simulink library "csu_egm_estimated_gravity_model_lib"  (R2014b)
settings: Solver=ode45  StartTime=0.0  StopTime=10.0  RelTol=1e-3
undefined symbols (not defined in the file or in its folder): central_body_flattening, central_body_gravity_mu, gsh_a, gsh_b, gsh_e, gsh_ep, magnitude
libraries: util_quat_lib x7, util_common_lib x3, util_fsw_frame_rotation_lib x2
settings Model: Creator=escrane  LastModifiedBy=escrane

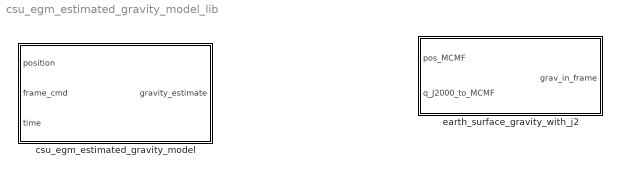
== system csu_egm_estimated_gravity_model_lib ==
  csu_egm_estimated_gravity_model : Subsystem
  earth_surface_gravity_with_j2 : Subsystem

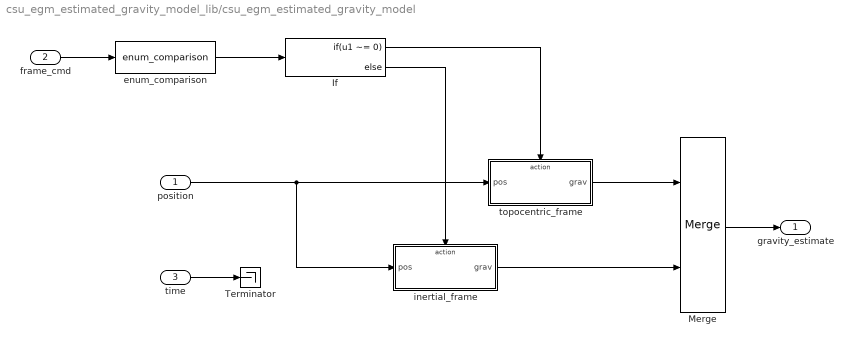
== system csu_egm_estimated_gravity_model_lib/csu_egm_estimated_gravity_model ==
  position : Inport
  frame_cmd : Inport  Port=2
  time : Inport  Port=3
  If : If  IfExpression=u1 ~= 0
  Merge : Merge
  Terminator : Terminator
  enum_comparison : util_common_lib/enum_comparison  comparison_type===
  inertial_frame : Subsystem
  topocentric_frame : Subsystem
  gravity_estimate : Outport
  wires:
  position/1 -> inertial_frame/1(pos), topocentric_frame/1(pos)
  frame_cmd/1 -> enum_comparison/1
  enum_comparison/1 -> If/1
  If/1 -> topocentric_frame/Action
  If/2 -> inertial_frame/Action
  topocentric_frame/1(grav) -> Merge/1
  inertial_frame/1(grav) -> Merge/2
  Merge/1 -> gravity_estimate/1
  time/1 -> Terminator/1

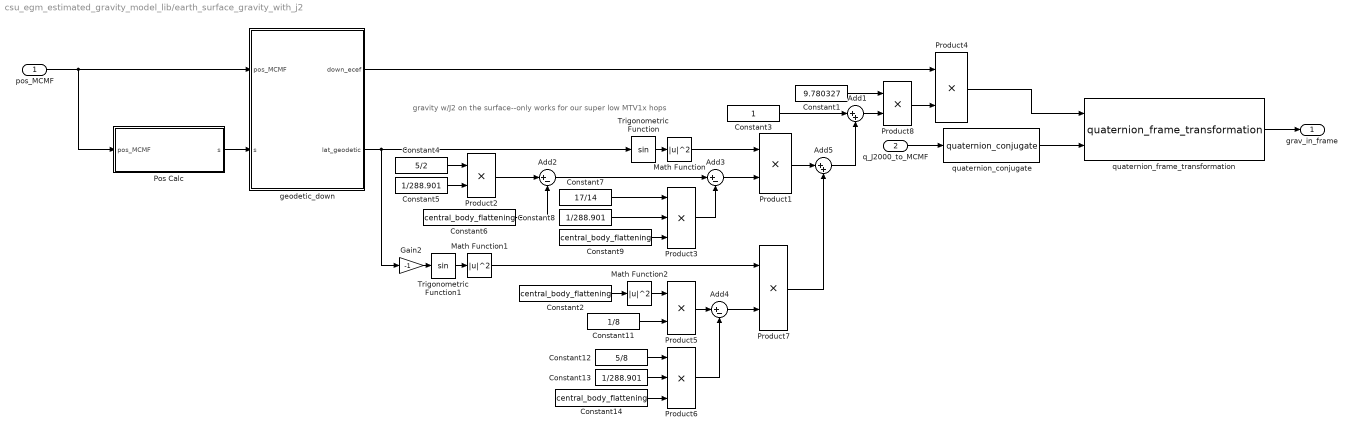
== system csu_egm_estimated_gravity_model_lib/earth_surface_gravity_with_j2 ==
  note: gravity w/J2 on the surface--only works for our super low MTV1x hops
  pos_MCMF : Inport
  q_J2000_to_MCMF : Inport  Port=2
  Add1 : Sum  Inputs=|++
  Add2 : Sum  Inputs=|+-
  Add3 : Sum  Inputs=|+-
  Add4 : Sum  Inputs=|+-
  Add5 : Sum  Inputs=|++
  Constant1 : Constant  Value=9.780327
  Constant11 : Constant  Value=1/8
  Constant12 : Constant  Value=5/8
  Constant13 : Constant  Value=1/288.901
  Constant{2,6,9,14} (4 alike) : Constant  Value=central_body_flattening
  Constant3 : Constant
  Constant4 : Constant  Value=5/2
  Constant5 : Constant  Value=1/288.901
  Constant7 : Constant  Value=17/14
  Constant8 : Constant  Value=1/288.901
  Gain2 : Gain  Gain=-1
  Math Function : Math  Operator=magnitude^2  SaturateOnIntegerOverflow=on
  Math Function1 : Math  Operator=magnitude^2  SaturateOnIntegerOverflow=on
  Math Function2 : Math  Operator=magnitude^2  SaturateOnIntegerOverflow=on
  Pos Calc : Subsystem
  Product{1..2,4..5,7..8} (6 alike) : Product
  Product3 : Product  Inputs=3
  Product6 : Product  Inputs=3
  Trigonometric Function : Trigonometry
  Trigonometric Function1 : Trigonometry
  geodetic_down : Subsystem
  quaternion_conjugate : util_quat_lib/quaternion_conjugate  SystemSampleTime=-1
  quaternion_frame_transformation : util_quat_lib/quaternion_frame_transformation  SystemSampleTime=-1
  grav_in_frame : Outport
  wires:
  quaternion_frame_transformation/1 -> grav_in_frame/1
  Product4/1 -> quaternion_frame_transformation/1
  quaternion_conjugate/1 -> quaternion_frame_transformation/2
  q_J2000_to_MCMF/1 -> quaternion_conjugate/1
  Pos Calc/1(s) -> geodetic_down/2(s)
  pos_MCMF/1 -> Pos Calc/1(pos_MCMF), geodetic_down/1(pos_MCMF)
  Constant3/1 -> Add1/1
  Trigonometric Function/1 -> Math Function/1
  Trigonometric Function1/1 -> Math Function1/1
  geodetic_down/2(lat_geodetic) -> Gain2/1, Trigonometric Function/1
  Gain2/1 -> Trigonometric Function1/1
  Constant4/1 -> Product2/1
  Constant5/1 -> Product2/2
  Product2/1 -> Add2/1
  Constant6/1 -> Add2/2
  Constant7/1 -> Product3/1
  Constant8/1 -> Product3/2
  Constant9/1 -> Product3/3
  Add2/1 -> Add3/1
  Product3/1 -> Add3/2
  Math Function/1 -> Product1/1
  Add3/1 -> Product1/2
  Constant2/1 -> Math Function2/1
  Math Function2/1 -> Product5/1
  Constant11/1 -> Product5/2
  Constant12/1 -> Product6/1
  Constant13/1 -> Product6/2
  Constant14/1 -> Product6/3
  Product5/1 -> Add4/1
  Product6/1 -> Add4/2
  Add4/1 -> Product7/2
  Math Function1/1 -> Product7/1
  Product1/1 -> Add5/1
  Product7/1 -> Add5/2
  Add5/1 -> Add1/2
  Add1/1 -> Product8/2
  Constant1/1 -> Product8/1
  Product8/1 -> Product4/2
  geodetic_down/1(down_ecef) -> Product4/1

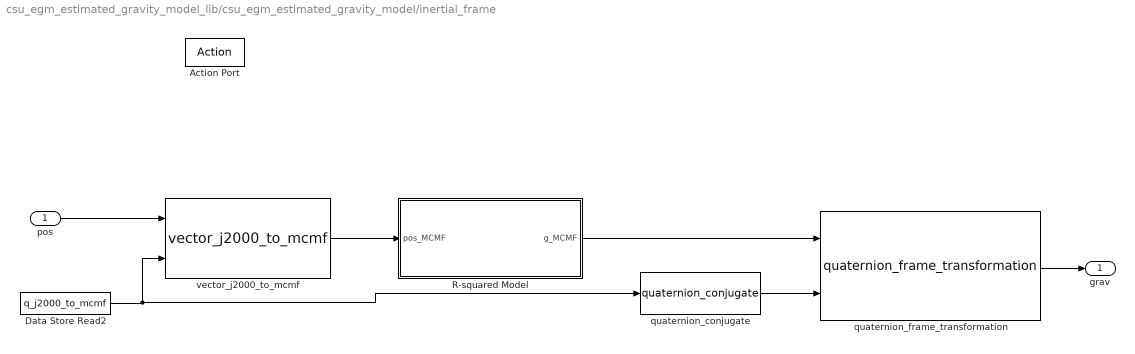
== system csu_egm_estimated_gravity_model_lib/csu_egm_estimated_gravity_model/inertial_frame ==
  pos : Inport
  Action Port : ActionPort
  Data Store Read2 : DataStoreRead  DataStoreName=q_j2000_to_mcmf
  R-squared Model : Subsystem
  quaternion_conjugate : util_quat_lib/quaternion_conjugate  SystemSampleTime=-1
  quaternion_frame_transformation : util_quat_lib/quaternion_frame_transformation  SystemSampleTime=-1
  vector_j2000_to_mcmf : util_fsw_frame_rotation_lib/vector_j2000_to_mcmf  SystemSampleTime=-1
  grav : Outport
  wires:
  R-squared Model/1(g_MCMF) -> quaternion_frame_transformation/1
  quaternion_conjugate/1 -> quaternion_frame_transformation/2
  pos/1 -> vector_j2000_to_mcmf/1
  quaternion_frame_transformation/1 -> grav/1
  Data Store Read2/1 -> vector_j2000_to_mcmf/2, quaternion_conjugate/1
  vector_j2000_to_mcmf/1 -> R-squared Model/1(pos_MCMF)

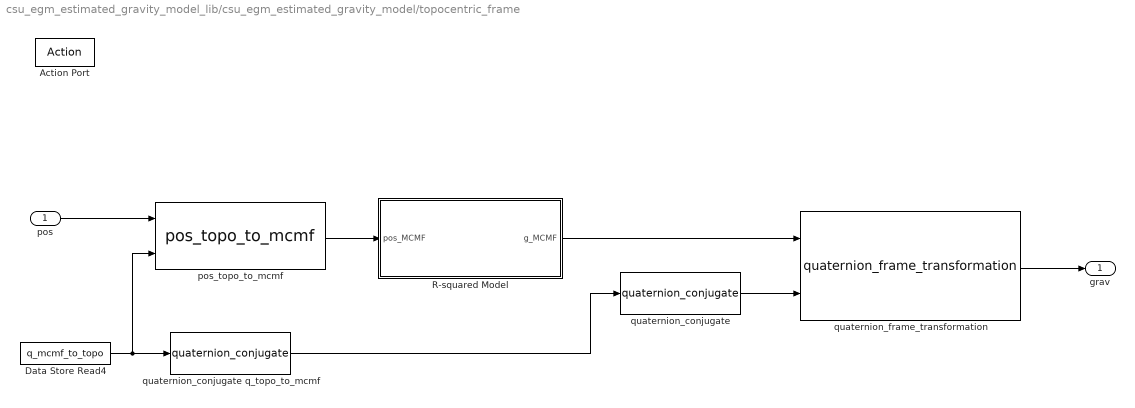
== system csu_egm_estimated_gravity_model_lib/csu_egm_estimated_gravity_model/topocentric_frame ==
  pos : Inport
  Action Port : ActionPort
  Data Store Read4 : DataStoreRead  DataStoreName=q_mcmf_to_topo
  R-squared Model : Subsystem
  pos_topo_to_mcmf : util_fsw_frame_rotation_lib/pos_topo_to_mcmf  SystemSampleTime=-1
  quaternion_conjugate : util_quat_lib/quaternion_conjugate  SystemSampleTime=-1
  quaternion_conjugate q_topo_to_mcmf : util_quat_lib/quaternion_conjugate  SystemSampleTime=-1
  quaternion_frame_transformation : util_quat_lib/quaternion_frame_transformation  SystemSampleTime=-1
  grav : Outport
  wires:
  R-squared Model/1(g_MCMF) -> quaternion_frame_transformation/1
  quaternion_conjugate/1 -> quaternion_frame_transformation/2
  quaternion_frame_transformation/1 -> grav/1
  pos_topo_to_mcmf/1 -> R-squared Model/1(pos_MCMF)
  pos/1 -> pos_topo_to_mcmf/1
  Data Store Read4/1 -> quaternion_conjugate q_topo_to_mcmf/1, pos_topo_to_mcmf/2
  quaternion_conjugate q_topo_to_mcmf/1 -> quaternion_conjugate/1

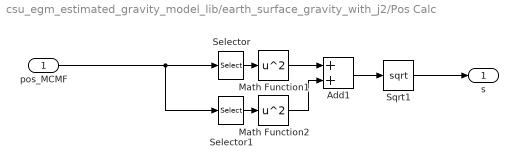
== system csu_egm_estimated_gravity_model_lib/earth_surface_gravity_with_j2/Pos Calc ==
  pos_MCMF : Inport
  Add1 : Sum
  Math Function1 : Math  Operator=square  SaturateOnIntegerOverflow=on
  Math Function2 : Math  Operator=square  SaturateOnIntegerOverflow=on
  Selector : Selector  InputPortWidth=3  Indices=[1]
  Selector1 : Selector  InputPortWidth=3  Indices=[2]
  Sqrt1 : Sqrt  SaturateOnIntegerOverflow=on
  s : Outport
  wires:
  pos_MCMF/1 -> Selector1/1, Selector/1
  Selector/1 -> Math Function1/1
  Selector1/1 -> Math Function2/1
  Add1/1 -> Sqrt1/1
  Sqrt1/1 -> s/1
  Math Function1/1 -> Add1/1
  Math Function2/1 -> Add1/2

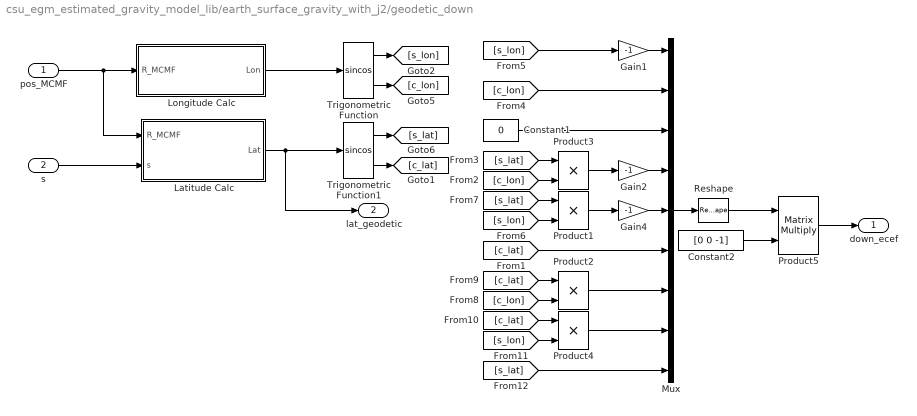
== system csu_egm_estimated_gravity_model_lib/earth_surface_gravity_with_j2/geodetic_down ==
  pos_MCMF : Inport
  s : Inport  Port=2
  Constant1 : Constant  Value=0
  Constant2 : Constant  Value=[0 0 -1]
  Gain1 : Gain  Gain=-1
  Gain2 : Gain  Gain=-1
  Gain4 : Gain  Gain=-1
  Latitude Calc : Subsystem
  Longitude Calc : Subsystem
  Mux : Mux  Inputs=9
  Product{1..4} (4 alike) : Product  RndMeth=Zero
  Product5 : Product  Multiplication=Matrix(*)  RndMeth=Zero
  Reshape : Reshape  OutputDimensionality=Customize  OutputDimensions=[3,3]
  Trigonometric Function : Trigonometry  Operator=sincos
  Trigonometric Function1 : Trigonometry  Operator=sincos
  down_ecef : Outport
  lat_geodetic : Outport  Port=2
  wires:
  Constant2/1 -> Product5/2
  Reshape/1 -> Product5/1
  Mux/1 -> Reshape/1
  [s_lat] -> Mux/9
  [s_lon] -> Product4/2
  Product4/1 -> Mux/8
  [c_lat] -> Product4/1
  [c_lon] -> Product2/2
  Product2/1 -> Mux/7
  [c_lat] -> Product2/1
  [c_lat] -> Mux/6
  Gain4/1 -> Mux/5
  Product1/1 -> Gain4/1
  [s_lon] -> Product1/2
  [s_lat] -> Product1/1
  Gain2/1 -> Mux/4
  Product3/1 -> Gain2/1
  [c_lon] -> Product3/2
  [s_lat] -> Product3/1
  Constant1/1 -> Mux/3
  [c_lon] -> Mux/2
  [s_lon] -> Gain1/1
  Gain1/1 -> Mux/1
  Trigonometric Function1/2 -> [c_lat]
  Trigonometric Function1/1 -> [s_lat]
  Trigonometric Function/2 -> [c_lon]
  Trigonometric Function/1 -> [s_lon]
  pos_MCMF/1 -> Latitude Calc/1(R_MCMF), Longitude Calc/1(R_MCMF)
  Latitude Calc/1(Lat) -> lat_geodetic/1, Trigonometric Function1/1
  Longitude Calc/1(Lon) -> Trigonometric Function/1
  Product5/1 -> down_ecef/1
  s/1 -> Latitude Calc/2(s)

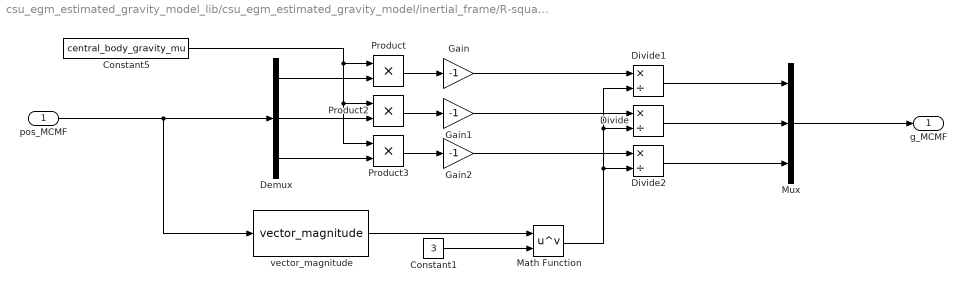
== system csu_egm_estimated_gravity_model_lib/csu_egm_estimated_gravity_model/inertial_frame/R-squared Model ==
  pos_MCMF : Inport
  Constant1 : Constant  Value=3
  Constant5 : Constant  Value=central_body_gravity_mu
  Demux : Demux  Outputs=3
  Divide : Product  Inputs=*/
  Divide1 : Product  Inputs=*/
  Divide2 : Product  Inputs=*/
  Gain : Gain  Gain=-1
  Gain1 : Gain  Gain=-1
  Gain2 : Gain  Gain=-1
  Math Function : Math  Operator=pow  SaturateOnIntegerOverflow=on
  Mux : Mux  Inputs=3
  Product : Product  RndMeth=Zero
  Product2 : Product  RndMeth=Zero
  Product3 : Product  RndMeth=Zero
  vector_magnitude : util_common_lib/vector_magnitude  SystemSampleTime=-1
  g_MCMF : Outport
  wires:
  pos_MCMF/1 -> Demux/1, vector_magnitude/1
  Constant1/1 -> Math Function/2
  Math Function/1 -> Divide2/2, Divide/2, Divide1/2
  vector_magnitude/1 -> Math Function/1
  Divide2/1 -> Mux/3
  Divide/1 -> Mux/2
  Divide1/1 -> Mux/1
  Gain2/1 -> Divide2/1
  Gain1/1 -> Divide/1
  Gain/1 -> Divide1/1
  Product/1 -> Gain/1
  Product2/1 -> Gain1/1
  Product3/1 -> Gain2/1
  Constant5/1 -> Product/1, Product2/1, Product3/1
  Demux/2 -> Product2/2
  Demux/1 -> Product/2
  Demux/3 -> Product3/2
  Mux/1 -> g_MCMF/1

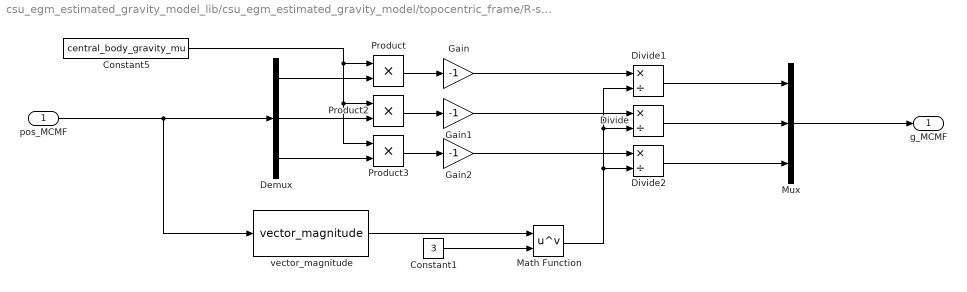
== system csu_egm_estimated_gravity_model_lib/csu_egm_estimated_gravity_model/topocentric_frame/R-squared Model ==
  pos_MCMF : Inport
  Constant1 : Constant  Value=3
  Constant5 : Constant  Value=central_body_gravity_mu
  Demux : Demux  Outputs=3
  Divide : Product  Inputs=*/
  Divide1 : Product  Inputs=*/
  Divide2 : Product  Inputs=*/
  Gain : Gain  Gain=-1
  Gain1 : Gain  Gain=-1
  Gain2 : Gain  Gain=-1
  Math Function : Math  Operator=pow  SaturateOnIntegerOverflow=on
  Mux : Mux  Inputs=3
  Product : Product  RndMeth=Zero
  Product2 : Product  RndMeth=Zero
  Product3 : Product  RndMeth=Zero
  vector_magnitude : util_common_lib/vector_magnitude  SystemSampleTime=-1
  g_MCMF : Outport
  wires:
  pos_MCMF/1 -> Demux/1, vector_magnitude/1
  Constant1/1 -> Math Function/2
  Math Function/1 -> Divide2/2, Divide/2, Divide1/2
  vector_magnitude/1 -> Math Function/1
  Divide2/1 -> Mux/3
  Divide/1 -> Mux/2
  Divide1/1 -> Mux/1
  Gain2/1 -> Divide2/1
  Gain1/1 -> Divide/1
  Gain/1 -> Divide1/1
  Product/1 -> Gain/1
  Product2/1 -> Gain1/1
  Product3/1 -> Gain2/1
  Constant5/1 -> Product/1, Product2/1, Product3/1
  Demux/2 -> Product2/2
  Demux/1 -> Product/2
  Demux/3 -> Product3/2
  Mux/1 -> g_MCMF/1

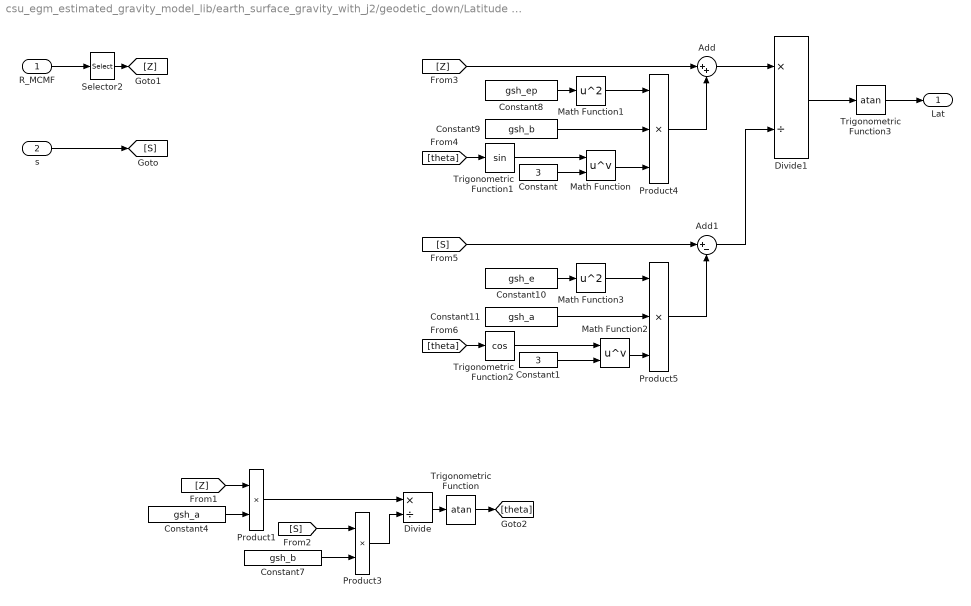
== system csu_egm_estimated_gravity_model_lib/earth_surface_gravity_with_j2/geodetic_down/Latitude Calc ==
  R_MCMF : Inport
  s : Inport  Port=2
  Add : Sum  Inputs=|++
  Add1 : Sum  Inputs=|+-
  Constant : Constant  Value=3
  Constant1 : Constant  Value=3
  Constant10 : Constant  Value=gsh_e
  Constant11 : Constant  Value=gsh_a
  Constant4 : Constant  Value=gsh_a
  Constant7 : Constant  Value=gsh_b
  Constant8 : Constant  Value=gsh_ep
  Constant9 : Constant  Value=gsh_b
  Divide : Product  Inputs=*/
  Divide1 : Product  Inputs=*/
  Math Function : Math  Operator=pow  SaturateOnIntegerOverflow=on
  Math Function1 : Math  Operator=square  SaturateOnIntegerOverflow=on
  Math Function2 : Math  Operator=pow  SaturateOnIntegerOverflow=on
  Math Function3 : Math  Operator=square  SaturateOnIntegerOverflow=on
  Product1 : Product
  Product3 : Product
  Product4 : Product  Inputs=3
  Product5 : Product  Inputs=3
  Selector2 : Selector  InputPortWidth=3  Indices=[3]
  Trigonometric Function : Trigonometry  Operator=atan
  Trigonometric Function1 : Trigonometry
  Trigonometric Function2 : Trigonometry  Operator=cos
  Trigonometric Function3 : Trigonometry  Operator=atan
  Lat : Outport
  wires:
  R_MCMF/1 -> Selector2/1
  s/1 -> [S]
  Selector2/1 -> [Z]
  Constant4/1 -> Product1/2
  [Z] -> Product1/1
  Product1/1 -> Divide/1
  Constant7/1 -> Product3/2
  [S] -> Product3/1
  Product3/1 -> Divide/2
  Divide/1 -> Trigonometric Function/1
  [Z] -> Add/1
  Constant8/1 -> Math Function1/1
  Math Function1/1 -> Product4/1
  Constant9/1 -> Product4/2
  Trigonometric Function1/1 -> Math Function/1
  Constant/1 -> Math Function/2
  Math Function/1 -> Product4/3
  Product4/1 -> Add/2
  Add/1 -> Divide1/1
  [S] -> Add1/1
  Constant10/1 -> Math Function3/1
  Math Function3/1 -> Product5/1
  Constant11/1 -> Product5/2
  Trigonometric Function2/1 -> Math Function2/1
  Constant1/1 -> Math Function2/2
  Math Function2/1 -> Product5/3
  Product5/1 -> Add1/2
  Add1/1 -> Divide1/2
  Divide1/1 -> Trigonometric Function3/1
  Trigonometric Function3/1 -> Lat/1
  Trigonometric Function/1 -> [theta]
  [theta] -> Trigonometric Function1/1
  [theta] -> Trigonometric Function2/1

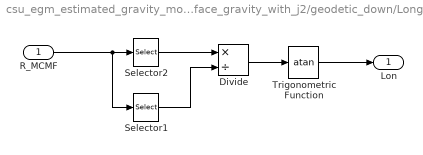
== system csu_egm_estimated_gravity_model_lib/earth_surface_gravity_with_j2/geodetic_down/Longitude Calc ==
  R_MCMF : Inport
  Divide : Product  Inputs=*/
  Selector1 : Selector  InputPortWidth=3  Indices=[1]
  Selector2 : Selector  InputPortWidth=3  Indices=[2]
  Trigonometric Function : Trigonometry  Operator=atan
  Lon : Outport
  wires:
  R_MCMF/1 -> Selector1/1, Selector2/1
  Selector2/1 -> Divide/1
  Selector1/1 -> Divide/2
  Divide/1 -> Trigonometric Function/1
  Trigonometric Function/1 -> Lon/1
